simulink model "quadrotor_control"  (R2020a)
settings: Solver=ode1  StartTime=0.0  StopTime=10.0  RelTol=1e-3
settings Model: Creator=lucas  LastModifiedBy=lucas

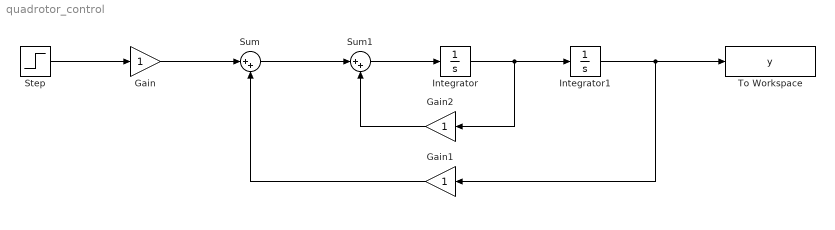
== system quadrotor_control ==
  Gain : Gain
  Gain1 : Gain
  Gain2 : Gain
  Integrator : Integrator
  Integrator1 : Integrator
  Step : Step  Time=0  SampleTime=0
  Sum : Sum  Inputs=|++
  Sum1 : Sum  Inputs=|++
  To Workspace : ToWorkspace  VariableName=y  SaveFormat=Structure With Time  SampleTime=-1
  wires:
  Step/1 -> Gain/1
  Gain/1 -> Sum/1
  Sum/1 -> Sum1/1
  Integrator/1 -> Gain2/1, Integrator1/1
  Sum1/1 -> Integrator/1
  Gain2/1 -> Sum1/2
  Integrator1/1 -> Gain1/1, To Workspace/1
  Gain1/1 -> Sum/2
